simulink model "line_equation_mask"  (R2021a)
settings: Solver=VariableStepAuto  StartTime=0.0  StopTime=10.0  RelTol=1e-3
settings Model: Creator=YasserNet  LastModifiedBy=YasserNet

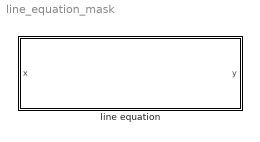
== system line_equation_mask ==
  line equation : Subsystem  mask{m=0, b=0}
      mask prompts: m "slope"; b "intersection"
      mask DialogControl DescGroupVar Prompt: line equation
      mask Display:
      | x=linspace(0,1,100);
      | t=linspace(0,1,100);
      | plot(x,t)

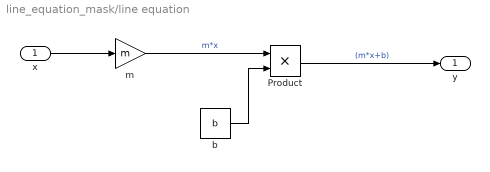
== system line_equation_mask/line equation ==
  x : Inport
  Product : Product
  b : Constant  Value=b
  m : Gain  Gain=m
  y : Outport
  wires:
  b/1 -> Product/2
  x/1 -> m/1
  Product/1 -> y/1  "(m*x+b)"
  m/1 -> Product/1  "m*x"
